simulink model "MajorProject_2"  (Simulink 7.3)
settings: Solver=ode45  StartTime=0.0  StopTime=0.08  RelTol=1e-3
libraries: powerlib x19, powerlib_extras x1
settings Model: Creator=win7  LastModifiedBy=win7

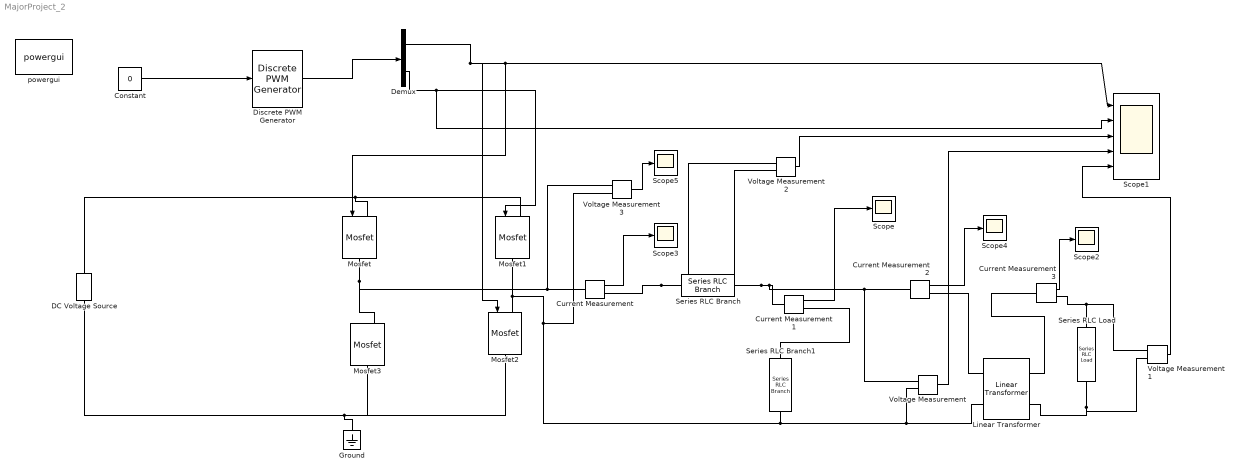
== system MajorProject_2 ==
  Constant : Constant  Value=0  OutDataType=fixdt(1, 16)  OutScaling=2^0
  Current Measurement{,1..3} (4 alike) : powerlib/Measurements/Current Measurement  DialogController=POWERSYS.PowerSysDialog  SystemSampleTime=-1  PhasorSimulation=off  OutputType=Complex  PSBequivalent=0
  DC Voltage Source : powerlib/Electrical Sources/DC Voltage Source  DialogController=POWERSYS.PowerSysDialog  SystemSampleTime=-1  Amplitude=120  Measurements=None
  Demux : Demux  Outputs=2
  Discrete PWM Generator : powerlib_extras/Discrete  Control Blocks/Discrete PWM Generator  DialogController=POWERSYS.PowerSysDialog  SystemSampleTime=-1  GeneratorMode="1-arm  bridge (2 pulses)"  Fc=50000  Ts=5e-6  Internal=off  mIndex=0.4  Freq=60  Phase=0
  Ground : powerlib/Elements/Ground  DialogController=POWERSYS.PowerSysDialog  PhysicalDomain=powersysdomain  SubClassName=unknown  LeftPortType=p1  RightPortType=p1  LConnTagsString=a
  Linear Transformer : powerlib/Elements/Linear Transformer  DialogController=POWERSYS.PowerSysDialog  PhysicalDomain=powersysdomain  SubClassName=unknown  LeftPortType=p1  RightPortType=p1  LConnTagsString=a|b  RConnTagsString=A|B  UNITS=pu  NominalPower=[ 250e6 60 ]  winding1="[ 735e3  0.002  0.08 ]"  winding2="[ 315e3  0.002  0.08 ]"  ThreeWindings=off  winding3=[ 315e3 0.002 0.08 ]  RmLm=[ 500 500 ]  Measurements=None  DataType=off
  Mosfet{,1..3} (4 alike) : powerlib/Power Electronics/Mosfet  DialogController=POWERSYS.PowerSysDialog  SystemSampleTime=-1  Ron=0.1  Lon=0  Rd=0.01  Vfd=0  IC=0  Rs=1e5  Cs=inf  Measurements=off
  Scope{,2..5} (5 alike) : Scope
      Scope2 settings: SaveName=ScopeData2
      Scope3 settings: YMin=-40  YMax=40  SaveName=ScopeData3
      Scope4 settings: SaveName=ScopeData4
      Scope5 settings: YMin=-180  YMax=180  SaveName=ScopeData5
  Scope1 : Scope  NumInputPorts=5
      settings: TimeRange=0.003499999999999948  YMin=0~0~-500~-500~-0.75  YMax=1~1~600~500~0.75
  Series RLC Branch : powerlib/Elements/Series RLC Branch  DialogController=POWERSYS.PowerSysDialog  PhysicalDomain=powersysdomain  SubClassName=unknown  LeftPortType=p1  RightPortType=p1  LConnTagsString=__new0  RConnTagsString=__new0  BranchType=C  Resistance=1  Inductance=1e-3  SetiL0=off  InitialCurrent=0  Capacitance=2e-7  Setx0=off  InitialVoltage=0  Measurements=None
  Series RLC Branch1 : powerlib/Elements/Series RLC Branch  DialogController=POWERSYS.PowerSysDialog  PhysicalDomain=powersysdomain  SubClassName=unknown  LeftPortType=p1  RightPortType=p1  LConnTagsString=__new0  RConnTagsString=__new0  BranchType=L  Resistance=1  Inductance=4e-5  SetiL0=off  InitialCurrent=0  Capacitance=1e-6  Setx0=off  InitialVoltage=0  Measurements=None
  Series RLC Load : powerlib/Elements/Series RLC Load  DialogController=POWERSYS.PowerSysDialog  PhysicalDomain=powersysdomain  SubClassName=unknown  LeftPortType=p1  RightPortType=p1  LConnTagsString=a  RConnTagsString=__new0  NominalVoltage=1000  NominalFrequency=50  ActivePower=5000  InductivePower=0  CapacitivePower=0  Setx0=off  InitialVoltage=0  SetiL0=off  InitialCurrent=0  Measurements=None
  Voltage Measurement{,1..3} (4 alike) : powerlib/Measurements/Voltage Measurement  DialogController=POWERSYS.PowerSysDialog  SystemSampleTime=-1  PhasorSimulation=off  OutputType=Complex  PSBequivalent=0
  powergui : powerlib/powergui  Priority=1  SystemSampleTime=-1  SimulationMode=Continuous  SampleTime=50e-6  frequency=60  SPID=off  DisableSnubberDevices=off  DisableRonSwitches=off  DisableVfSwitches=off  SwTol=0  Interpol=off  frequencyindice=0  echomessages=off  HookPort=off  DisplayEquations=off  FunctionMessages=off  EnableUseOfTLC=off  x0status=blocks  RestoreLinks=warning  Frange=[0:2:500]  Ylog=off  Xlog=on  ShowGrid=off  save=off  variable=ZData  ZoomFFT=on  StartTime=0.0  cycles=1  DisplayStyle=1  fundamental=60  FreqAxis=off  MaxFrequency=1000  frequencyindicesteady=1  RmsSteady=1  display=off  Ts=0  methode=off
  wires:
  Constant/1 -> Discrete PWM Generator/1
  Demux/1 -> Mosfet2/1, Mosfet/1, Scope1/1
  Demux/2 -> Mosfet1/1, Scope1/2
  Current Measurement1/1 -> Scope/1
  Current Measurement3/1 -> Scope2/1
  Current Measurement/1 -> Scope3/1
  Voltage Measurement2/1 -> Scope1/3
  Discrete PWM Generator/1 -> Demux/1
  Voltage Measurement1/1 -> Scope1/5
  Voltage Measurement/1 -> Scope1/4
  Current Measurement2/1 -> Scope4/1
  Voltage Measurement3/1 -> Scope5/1
  connections:
  Mosfet1/RConn1 -- Mosfet2/LConn1 -- Linear Transformer/LConn2 -- Voltage Measurement/LConn2 -- Series RLC Branch1/RConn1 -- Voltage Measurement3/LConn2
  Current Measurement/LConn1 -- Voltage Measurement3/LConn1 -- Mosfet/RConn1 -- Mosfet3/LConn1
  Ground/LConn1 -- Mosfet3/RConn1 -- Mosfet2/RConn1 -- DC Voltage Source/LConn1
  DC Voltage Source/RConn1 -- Mosfet1/LConn1 -- Mosfet/LConn1
  Current Measurement/RConn1 -- Series RLC Branch/LConn1 -- Voltage Measurement2/LConn1
  Current Measurement1/LConn1 -- Current Measurement2/LConn1 -- Voltage Measurement/LConn1 -- Series RLC Branch/RConn1 -- Voltage Measurement2/LConn2
  Current Measurement1/RConn1 -- Series RLC Branch1/LConn1
  Current Measurement2/RConn1 -- Linear Transformer/LConn1
  Linear Transformer/RConn1 -- Current Measurement3/LConn1
  Series RLC Load/RConn1 -- Current Measurement3/RConn1 -- Voltage Measurement1/LConn1
  Series RLC Load/LConn1 -- Linear Transformer/RConn2 -- Voltage Measurement1/LConn2
